simulink model "A4D_LQR"  (R2016a)
settings: Solver=VariableStepAuto  StartTime=0.0  StopTime=10.0  RelTol=1e-3
settings Model: Creator=kumabhi  LastModifiedBy=kumabhi

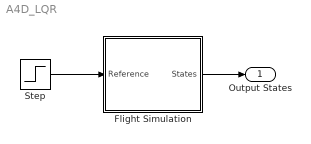
== system A4D_LQR ==
  Flight Simulation : Subsystem
      mask Display: image('/home/kumabhi/Documents/Courses/Thesis/plane-icon-vector-.jpg');
  Step : Step  After=1.0472  SampleTime=0
  Output States : Outport
  wires:
  Step/1 -> Flight Simulation/1(Reference)
  Flight Simulation/1(States) -> Output States/1

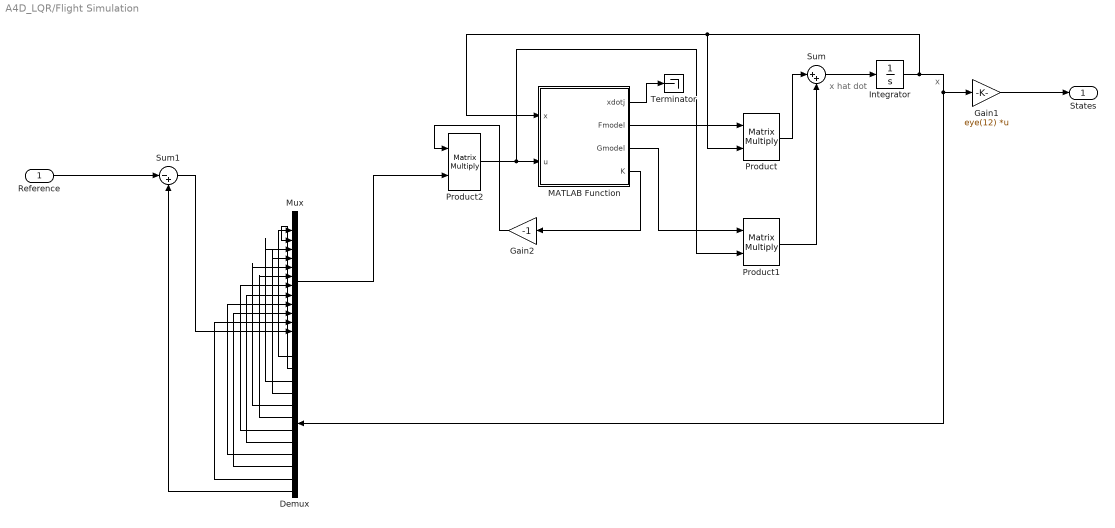
== system A4D_LQR/Flight Simulation ==
  note: x
  note: x hat dot
  Reference : Inport
  Demux : Demux  Outputs=12
  Gain1 : Gain  Gain=eye(12)  Multiplication=Matrix(K*u)
  Gain2 : Gain  Gain=-1
  Integrator : Integrator
  MATLAB Function : MATLAB Function  TreatAsAtomicUnit=on
  Mux : Mux  Inputs=12
  Product : Product  Multiplication=Matrix(*)
  Product1 : Product  Multiplication=Matrix(*)
  Product2 : Product  Multiplication=Matrix(*)
  Sum : Sum  Inputs=|++
  Sum1 : Sum  Inputs=|-+
  Terminator : Terminator
  States : Outport
  wires:
  Reference/1 -> Sum1/1
  Product1/1 -> Sum/2
  MATLAB Function/4(K) -> Gain2/1
  Gain2/1 -> Product2/1
  MATLAB Function/1(xdotj) -> Terminator/1
  Product/1 -> Sum/1
  MATLAB Function/3(Gmodel) -> Product1/1
  Sum/1 -> Integrator/1
  MATLAB Function/2(Fmodel) -> Product/1
  Product2/1 -> Product1/2, MATLAB Function/2(u)
  Gain1/1 -> States/1
  Integrator/1 -> Demux/1, Gain1/1, MATLAB Function/1(x), Product/2
  Demux/1 -> Mux/1
  Demux/2 -> Mux/2
  Demux/3 -> Mux/3
  Demux/4 -> Mux/4
  Demux/5 -> Mux/5
  Demux/6 -> Mux/6
  Demux/7 -> Mux/7
  Demux/8 -> Mux/8
  Demux/9 -> Mux/9
  Demux/10 -> Mux/10
  Demux/11 -> Mux/11
  Demux/12 -> Sum1/2
  Sum1/1 -> Mux/12
  Mux/1 -> Product2/2

== matlab function A4D_LQR/Flight Simulation/MATLAB Function ==
  data: xdotj output; x input; u input; Fmodel output; Gmodel output; K output
function[xdotj, Fmodel, Gmodel, K] = fcn(x, u)
%LINEARIZATION

thresh	=	[.1;.1;.1;.1;.1;.1;.1;.1;.1;.1;.1;.1;.1;.1;.1;.1];
xj		=	[x;u];
uTemp       =   u;  % 'numjac' modifies 'u'; reset 'u' after the call
xdotj       =   zeros(16,1);
xdotj		=	LinModel(0,xj);
coder.extrinsic('numjac');
dFdX        =   zeros(12,16);
[dFdX,fac]	=	numjac('LinModel',0,xj,xdotj,thresh,[],0);
u           =   uTemp;
% Gmodel      =   zeros(12,4);
Fmodel		=	dFdX(1:12,1:12)
Gmodel		=	dFdX(1:12,13:16)
Q = [0 0 0 0 0 0 0 0 0 0 0 0;
    0 0 0 0 0 0 0 0 0 0 0 0;
    0 0 0 0 0 0 0 0 0 0 0 0;
    0 0 0 0 0 0 0 0 0 0 0 0;
    0 0 0 0 0 0 0 0 0 0 0 0;
    0 0 0 0 0 0 0 0 0 0 0 0;
    0 0 0 0 0 0 0 0 0 0 0 0;
    0 0 0 0 0 0 0 0 0 0 0 0;
    0 0 0 0 0 0 0 0 0 0 0 0;
    0 0 0 0 0 0 0 0 0 10 0 0;
    0 0 0 0 0 0 0 0 0 0 10 0;
    0 0 0 0 0 0 0 0 0 0 0 10];
R = [1 0 0 0;
    0 1 0 0;
    0 0 1 0;
    0 0 0 1];
coder.extrinsic('lqr');
K   = zeros(4,12);
[K] = lqr(Fmodel, Gmodel, Q, R)
% save ('FmodelFile','Fmodel','TASms','hm','TrimAlphaDeg')
% save ('GmodelFile','Gmodel')
